simulink model "system_simulink"  (R2021b)
settings: Solver=ode45  StartTime=0.0  StopTime=20  RelTol=1e-3  EnableMultiTasking=on
undefined symbols (not defined in the file): K, static_compensator
libraries: simulink x1
settings Model: Creator=Cabral  LastModifiedBy=Mohammad masih
settings SolverCC: AlgebraicLoopSolver=TrustRegion
settings DataIOCC: LimitDataPoints=on  SaveFormat=Array  SignalLoggingSaveFormat=ModelDataLogs  ReturnWorkspaceOutputs=off
settings OptimizationCC: ExpressionDepthLimit=2147483647  InitFltsAndDblsToZero=on  LifeSpan=inf
settings DebuggingCC: SaveWithParameterizedLinksMsg=none  UnderspecifiedInitializationDetection=Classic  MergeDetectMultiDrivingBlocksExec=none  SignalResolutionControl=TryResolveAllWithWarning  SolverPrmCheckMsg=warning  MultiTaskDSMMsg=warning  MultiTaskCondExecSysMsg=none  FcnCallInpInsideContextMsg=warning  StateNameClashWarn=warning  SFUnexpectedBacktrackingDiag=warning  SFNoUnconditionalDefaultTransitionDiag=warning  SFExecutionAtInitializationDiag=none  SFMachineParentedDataDiag=warning  ArithmeticOperatorsInVariantConditions=warning
settings HardwareCC: ProdBitPerPointer=32  ProdBitPerSizeT=32  ProdBitPerPtrDiffT=32  ProdLargestAtomicFloat=None  ProdIntDivRoundTo=Undefined  ProdEndianess=Unspecified  ProdWordSize=32  ProdHWDeviceType=32-bit Generic
settings ModelReferenceCC: PropagateSignalLabelsOutOfModel=off
settings SFSimCC: SimUseLocalCustomCode=off  SimParseCustomCode=off  CustomCodeUndefinedFunction=UseInterfaceOnly
settings RTWCC: RTWUseLocalCustomCode=off
settings CodeAppCC: StateflowObjectComments=on
settings GRTTargetCC: TargetFcnLib=ansi_tfl_tmw.mat  TargetLangStandard=C89/C90 (ANSI)  CombineOutputUpdateFcns=off  GRTInterface=on
settings ConfigComp: CovMetricSettings=dw  CovSaveCumulativeToWorkspaceVar=on  CovSaveSingleToWorkspaceVar=on  CovExternalEMLEnable=off

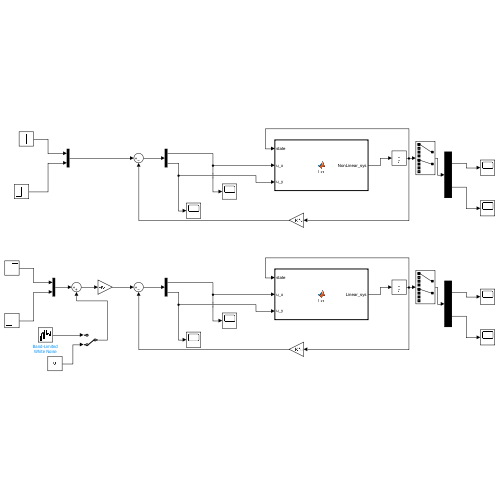
[thumbnail: Simulink's stored preview of the top-level diagram]
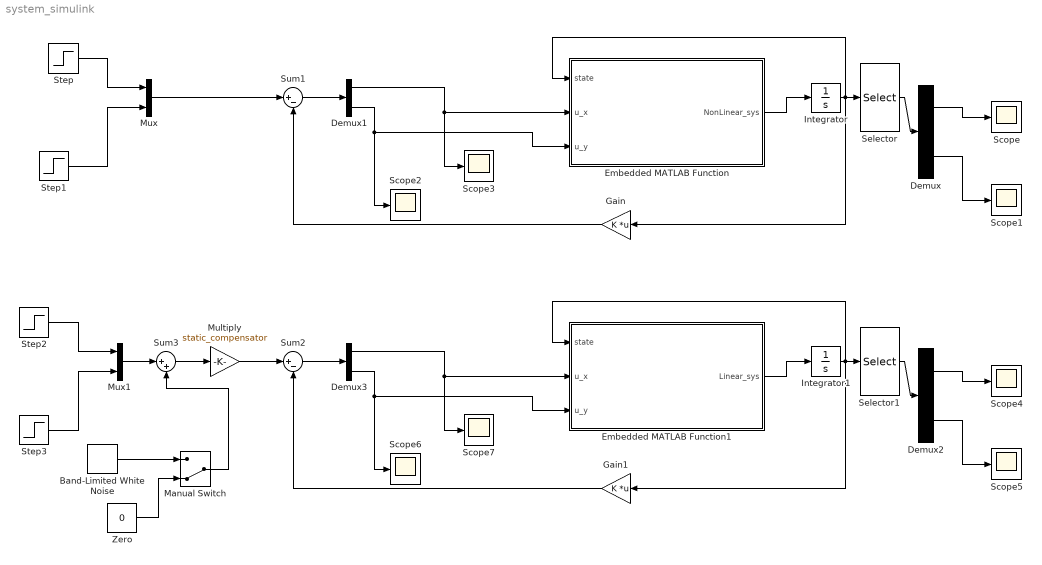
== system system_simulink ==
  Band-Limited White Noise : simulink/Sources/Band-Limited White Noise  Cov=[0.1]  Ts=0.1  seed=[23341]
  Demux{,1..3} (4 alike) : Demux  Outputs=[1 1]
  Embedded MATLAB Function : MATLAB Function  TreatAsAtomicUnit=on
  Embedded MATLAB Function1 : MATLAB Function  TreatAsAtomicUnit=on
  Gain : Gain  Gain=K  Multiplication=Matrix(K*u)
  Gain1 : Gain  Gain=K  Multiplication=Matrix(K*u)
  Integrator : Integrator  InitialCondition=[0 0 0 0 0 0 0 0]
  Integrator1 : Integrator  InitialCondition=[0 0 0 0 0 0 0 0]
  Manual Switch : ManualSwitch  CurrentSetting=0
  Multiply : Gain  Gain=static_compensator
  Mux : Mux  Inputs=2
  Mux1 : Mux  Inputs=2
  Scope{,1..7} (8 alike) : Scope
  Selector : Selector  InputPortWidth=8  IndexOptions=Index vector (dialog)  Indices=[1 5]  OutputSizes=1
  Selector1 : Selector  InputPortWidth=8  IndexOptions=Index vector (dialog)  Indices=[1 5]  OutputSizes=1
  Step{,1..3} (4 alike) : Step  SampleTime=0
  Sum1 : Sum  Inputs=|+-
  Sum2 : Sum  Inputs=|+-
  Sum3 : Sum  Inputs=|++
  Zero : Constant  Value=0  OutDataTypeStr=Inherit: Inherit via back propagation
  wires:
  Integrator/1 -> Gain/1, Selector/1, Embedded MATLAB Function/1(state)
  Selector/1 -> Demux/1
  Demux/2 -> Scope1/1
  Embedded MATLAB Function/1(NonLinear_sys) -> Integrator/1
  Demux/1 -> Scope/1
  Step/1 -> Mux/1
  Step1/1 -> Mux/2
  Sum1/1 -> Demux1/1
  Demux1/1 -> Scope3/1, Embedded MATLAB Function/2(u_x)
  Demux1/2 -> Scope2/1, Embedded MATLAB Function/3(u_y)
  Gain/1 -> Sum1/2
  Mux/1 -> Sum1/1
  Demux3/1 -> Scope7/1, Embedded MATLAB Function1/2(u_x)
  Demux2/1 -> Scope4/1
  Sum2/1 -> Demux3/1
  Gain1/1 -> Sum2/2
  Step3/1 -> Mux1/2
  Demux3/2 -> Scope6/1, Embedded MATLAB Function1/3(u_y)
  Integrator1/1 -> Gain1/1, Selector1/1, Embedded MATLAB Function1/1(state)
  Demux2/2 -> Scope5/1
  Selector1/1 -> Demux2/1
  Embedded MATLAB Function1/1(Linear_sys) -> Integrator1/1
  Step2/1 -> Mux1/1
  Multiply/1 -> Sum2/1
  Band-Limited White Noise/1 -> Manual Switch/1
  Sum3/1 -> Multiply/1
  Mux1/1 -> Sum3/1
  Manual Switch/1 -> Sum3/2
  Zero/1 -> Manual Switch/2

== matlab function system_simulink/Embedded MATLAB Function ==
  data: state input; u_x input; u_y input; NonLinear_sys output
function NonLinear_sys= fcn(state,u_x,u_y)
% constants
m = 0.11;
Ib = 1.76e-5;
rb = 0.02;

b = m/ (m + Ib/ rb^2)
g = 9.81;

x = state(1);
x_dot = state(2);
alfa = state(3);
alfa_dot = state(4);
y = state(5);
y_dot = state(6);
beta = state(7);
beta_dot = state(8);
if(alfa>1.57)
    alfa=1.57
    alfa_dot=0
end

if(beta>1.57)
    beta=1.57
    beta_dot=0
end
x_dot_dot = b*(x*alfa_dot*alfa_dot+alfa_dot*y*beta_dot-g*sin(alfa));
alpha_dot_dot = u_x;
y_dot_dot=b*(y*beta_dot*beta_dot+x*alfa_dot*beta_dot-g*sin(beta));
beta_dot_dot=u_y;

NonLinear_sys = [x_dot; x_dot_dot ;alfa_dot; alpha_dot_dot; y_dot ; y_dot_dot ; beta_dot ; beta_dot_dot];

== matlab function system_simulink/Embedded MATLAB Function1 ==
  data: state input; u_x input; u_y input; Linear_sys output
function Linear_sys= fcn(state,u_x,u_y)

A = [    0    1.0000         0         0         0         0         0         0;
         0         0   -7.0071         0         0         0         0         0;
         0         0         0    1.0000         0         0         0         0;
         0         0         0         0         0         0         0         0;
         0         0         0         0         0    1.0000         0         0;
         0         0         0         0         0         0   -7.0071         0;
         0         0         0         0         0         0         0    1.0000;
         0         0         0         0         0         0         0         0];
B=[  0     0;
     0     0;
     0     0;
     1     0;
     0     0;
     0     0;
     0     0;
     0     1];


Linear_sys = A*state+B*[u_x;u_y];
